simulink model "Vjezba3"  (R2017a)
settings: Solver=VariableStepAuto  StartTime=0.0  StopTime=10.0  RelTol=1e-3
settings Model: Creator=korisnik  LastModifiedBy=korisnik

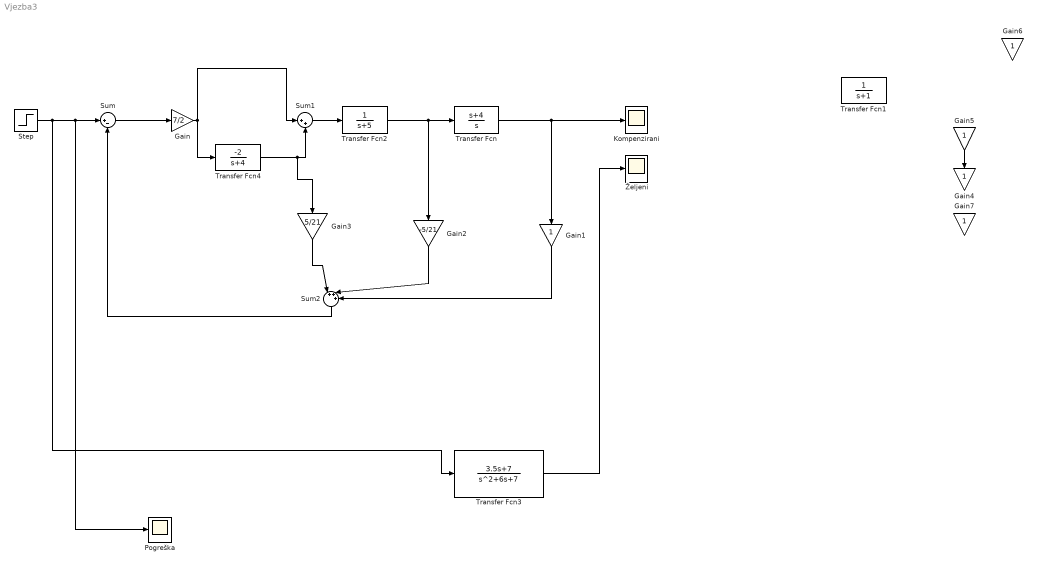
== system Vjezba3 ==
  Gain : Gain  Gain=7/2
  Gain{1,4..7} (5 alike) : Gain
  Gain2 : Gain  Gain=-5/21
  Gain3 : Gain  Gain=5/21
  Kompenzirani : Scope
  Pogreška : Scope
  Step : Step  SampleTime=0
  Sum : Sum  Inputs=|+-
  Sum1 : Sum  Inputs=|++
  Sum2 : Sum  Inputs=|+++
  Transfer Fcn : TransferFcn  Numerator=[1 4]  Denominator=[1 0]
  Transfer Fcn1 : TransferFcn  Denominator=[1 1]
  Transfer Fcn2 : TransferFcn  Denominator=[1 5]
  Transfer Fcn3 : TransferFcn  Numerator=[3.5 7]  Denominator=[1 6 7]
  Transfer Fcn4 : TransferFcn  Numerator=[-2]  Denominator=[1 4]
  Željeni : Scope
  wires:
  Step/1 -> Transfer Fcn3/1, Pogreška/1, Sum/1
  Sum/1 -> Gain/1
  Transfer Fcn2/1 -> Gain2/1, Transfer Fcn/1
  Gain/1 -> Transfer Fcn4/1, Sum1/1
  Transfer Fcn/1 -> Kompenzirani/1, Gain1/1
  Gain2/1 -> Sum2/2
  Gain1/1 -> Sum2/3
  Sum2/1 -> Sum/2
  Gain5/1 -> Gain4/1
  Transfer Fcn3/1 -> Željeni/1
  Sum1/1 -> Transfer Fcn2/1
  Transfer Fcn4/1 -> Gain3/1, Sum1/2
  Gain3/1 -> Sum2/1
